simulink library "uavGuidanceForEachMod"  (R2021a)
settings: Solver=VariableStepAuto  StartTime=0.0  StopTime=10.0  RelTol=1e-3
undefined symbols (not defined in the file or in its folder): convertStringsToChars, initialState, m
settings Model: Creator=fciriell  LastModifiedBy=fciriell

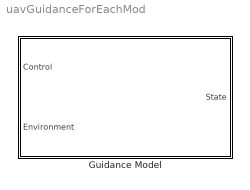
== system uavGuidanceForEachMod ==
  Guidance Model : Subsystem  mask(Guidance Model){ModelType=MultirotorGuidance, SpecifiedDataType=double, SimulateUsing=Code generation, InitialWorldPositionMultirotor=[0; 0; 0], InitialWorldVelocityMultirotor=[0; 0; 0], InitialEulerZYXMultirotor=[0; 0; 0], InitialBodyAngularRateRPYMultirotor=[0; 0; 0], InitialThrustMultirotor=0, InitialNorthFixedWing=0, InitialEastFixedWing=0, InitialHeightFixedWing=0, InitialAirSpeedFixedWing=0, InitialHeadingAngleFixedWing=0, InitialFlightPathAngleFixedWing=0, InitialRollAngleFixedWing=0, InitialRollAngleRateFixedWing=0, PDRollMultirotor=[3402.97,116.67], PDPitchMultirotor=[3402.97, 116.67], PYawRateMultirotor=1950, PThrustMultirotor=3900, MassMultirotor=m, PHeightFixedWing=3.9, PHeadingAngleFixedWing=3.9, PFlightPathAngleFixedWing=39, PDRollFixedWing=[3402.97, 116.67], PAirSpeedFixedWing=1, FlightPathAngleLimitsFixedWing=[-pi/2, pi/2], StateBusName='MultirotorGuidanceStateBus', ControlBusName='MultirotorGuidanceControlBus', EnvironmentBusName='MultirotorGuidanceEnvironmentBus', DataType=double}
      mask prompts: ModelType "uav:robotsluav:guidancemodelblock:ModelType"; SpecifiedDataType "uav:robotsluav:guidancemodelblock:DataType"; SimulateUsing "SystemBlock:MATLABSystem:SimulateUsing"; InitialWorldPositionMultirotor "uav:robotsluav:guidancemodelblock:WorldPosition"; InitialWorldVelocityMultirotor "uav:robotsluav:guidancemodelblock:WorldVelocity"; InitialEulerZYXMultirotor "uav:robotsluav:guidancemodelblock:EulerZYX"; InitialBodyAngularRateRPYMultirotor "uav:robotsluav:guidancemodelblock:BodyAngularRateRPY"; InitialThrustMultirotor "uav:robotsluav:guidancemodelblock:Thrust"; InitialNorthFixedWing "uav:robotsluav:guidancemodelblock:NorthPosition"; InitialEastFixedWing "uav:robotsluav:guidancemodelblock:EastPosition"; InitialHeightFixedWing "uav:robotsluav:guidancemodelblock:Height"; InitialAirSpeedFixedWing "uav:robotsluav:guidancemodelblock:AirSpeed"; InitialHeadingAngleFixedWing "uav:robotsluav:guidancemodelblock:HeadingAngle"; InitialFlightPathAngleFixedWing "uav:robotsluav:guidancemodelblock:FlightPathAngle"; InitialRollAngleFixedWing "uav:robotsluav:guidancemodelblock:RollAngle"; InitialRollAngleRateFixedWing "uav:robotsluav:guidancemodelblock:RollAngleRate"; PDRollMultirotor "uav:robotsluav:guidancemodelblock:PDRoll"; PDPitchMultirotor "uav:robotsluav:guidancemodelblock:PDPitch"; PYawRateMultirotor "uav:robotsluav:guidancemodelblock:PYawRate"; PThrustMultirotor "uav:robotsluav:guidancemodelblock:PThrust"; MassMultirotor "uav:robotsluav:guidancemodelblock:Mass"; PHeightFixedWing "uav:robotsluav:guidancemodelblock:PHeight"; PHeadingAngleFixedWing "uav:robotsluav:guidancemodelblock:PHeadingAngle"; PFlightPathAngleFixedWing "uav:robotsluav:guidancemodelblock:PFlightPathAngle"; PDRollFixedWing "uav:robotsluav:guidancemodelblock:PDRollAngle"; PAirSpeedFixedWing "uav:robotsluav:guidancemodelblock:PAirSpeed"; FlightPathAngleLimitsFixedWing "uav:robotsluav:guidancemodelblock:MinMaxFlightPathAngle"; StateBusName "uav:robotsluav:guidancemodelblock:StateBusName"; ControlBusName "uav:robotsluav:guidancemodelblock:ControlBusName"; EnvironmentBusName "uav:robotsluav:guidancemodelblock:EnvironmentBusName"; DataType "uav:robotsluav:guidancemodelblock:ResolvedDataType"
      mask help: uav:robotsluav:guidancemodelblock:Description
      mask init:
      | ModelName = gcb;
      | 
      | % Validate bus names
      | uav.sluav.internal.guidancemodel.mask.validateBusNames(gcb);
      | 
      | [stateDimension, initialState, UAVType, UAVDataType, UAVConfig] = ...
      |     uav.sluav.internal.guidancemodel.mask.initialize(ModelName, ModelType, gcb);
      mask Help: eval('helpview(fullfile(docroot, ''uav'', ''helptargets.map''), ''uavGuidanceModelBlock'')');
      mask TypeOptions ModelType: MultirotorGuidance | FixedWingGuidance
      mask Callback ModelType:
      | % Change mask dialog
      | uav.sluav.internal.guidancemodel.mask.modelTypeCallback(gcb);
      | 
      | % Create buses for the UAV block
      | uav.sluav.internal.guidancemodel.mask.createUAVBuses(gcb);
      mask Callback SpecifiedDataType:
      | if ~strcmp(get_param(gcb, 'SpecifiedDataType'), '<data type expression>')
      |     % Resolve input type
      |     uav.sluav.internal.guidancemodel.mask.dataTypeCallback(gcb);
      | 
      |     % Create buses for the UAV block
      |     uav.sluav.internal.guidancemodel.mask.createUAVBuses(gcb);
      | end
      mask TypeOptions SimulateUsing: ComputeDerivative/SimulateUsing | StateVector2Struct/SimulateUsing
      mask Callback StateBusName:
      | % Validate bus names
      | uav.sluav.internal.guidancemodel.mask.validateBusNames(gcb);
      | 
      | % Create buses for the UAV block
      | uav.sluav.internal.guidancemodel.mask.createUAVBuses(gcb);
      mask Callback ControlBusName:
      | % Validate bus names
      | uav.sluav.internal.guidancemodel.mask.validateBusNames(gcb);
      | 
      | % Create buses for the UAV block
      | uav.sluav.internal.guidancemodel.mask.createUAVBuses(gcb);
      mask Callback EnvironmentBusName:
      | % Validate bus names
      | uav.sluav.internal.guidancemodel.mask.validateBusNames(gcb);
      | 
      | % Create buses for the UAV block
      | uav.sluav.internal.guidancemodel.mask.createUAVBuses(gcb);
      mask DialogControl ModelType Prompt: Model Type:
      mask DialogControl SpecifiedDataType Prompt: Data Type:
      mask DialogControl SimulateUsing Prompt: Simulate using:
      mask DialogControl SimulateUsing Tooltip: SystemBlock:MATLABSystem:SimulateUsingDescription
      mask DialogControl InitialStateTab Prompt: uav:robotsluav:guidancemodelblock:InitialState
      mask DialogControl InitialWorldPositionMultirotor Prompt: World Position
      mask DialogControl InitialWorldVelocityMultirotor Prompt: World Velocity
      mask DialogControl InitialEulerZYXMultirotor Prompt: Euler Angles (ZYX)
      mask DialogControl InitialBodyAngularRateRPYMultirotor Prompt: Body Angular Rate
      mask DialogControl InitialThrustMultirotor Prompt: Thrust
      mask DialogControl InitialNorthFixedWing Prompt: North Position
      mask DialogControl InitialEastFixedWing Prompt: East Position
      mask DialogControl InitialHeightFixedWing Prompt: Height
      mask DialogControl InitialAirSpeedFixedWing Prompt: Air Speed
      mask DialogControl InitialHeadingAngleFixedWing Prompt: Heading Angle
      mask DialogControl InitialFlightPathAngleFixedWing Prompt: Flight Path Angle
      mask DialogControl InitialRollAngleFixedWing Prompt: Roll Angle
      mask DialogControl InitialRollAngleRateFixedWing Prompt: Roll Angular Velocity
      mask DialogControl ConfigurationTab Prompt: uav:robotsluav:guidancemodelblock:Configuration
      mask DialogControl PDRollMultirotor Prompt: PD Roll
      mask DialogControl PDPitchMultirotor Prompt: PD Pitch
      mask DialogControl PYawRateMultirotor Prompt: P YawRate
      mask DialogControl PThrustMultirotor Prompt: P Thrust
      mask DialogControl MassMultirotor Prompt: Mass
      mask DialogControl PHeightFixedWing Prompt: P Height
      mask DialogControl PHeadingAngleFixedWing Prompt: P Heading Angle
      mask DialogControl PFlightPathAngleFixedWing Prompt: P Flight Path Angle
      mask DialogControl PDRollFixedWing Prompt: PD Roll Angle
      mask DialogControl PAirSpeedFixedWing Prompt: P Air Speed
      mask DialogControl FlightPathAngleLimitsFixedWing Prompt: Min/Max Flight Path Angle
      mask DialogControl BusNameTab Prompt: uav:robotsluav:guidancemodelblock:InputOutputBusNames
      mask DialogControl StateBusName Prompt: State Bus Name
      mask DialogControl ControlBusName Prompt: Control Bus Name
      mask DialogControl EnvironmentBusName Prompt: Environment Bus Name
      mask DialogControl DataType Prompt: Resolved Data Type
      mask Display:
      | port_label('input', 1, 'Control')
      | port_label('input', 2, 'Environment')
      | port_label('output', 1, 'State')

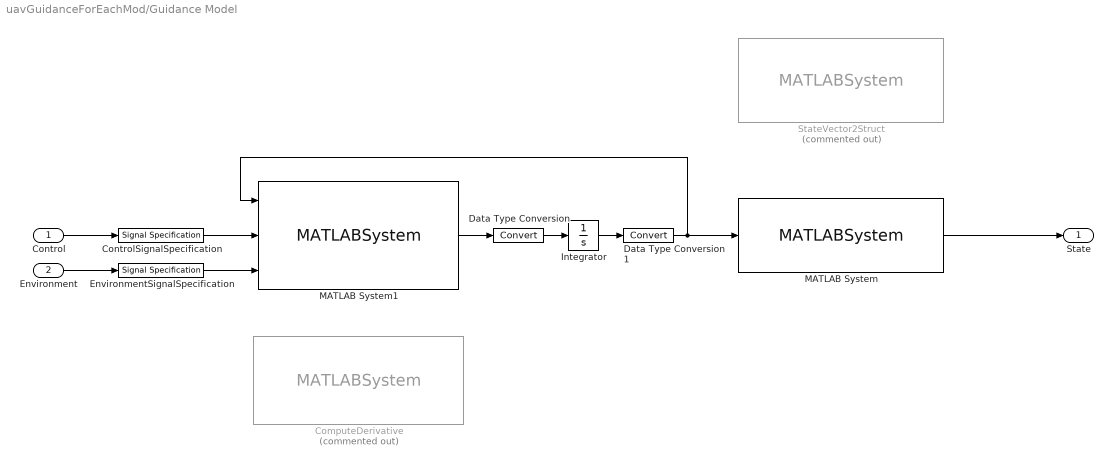
== system uavGuidanceForEachMod/Guidance Model ==
  Control : Inport
  Environment : Inport  Port=2
  ComputeDerivative : MATLABSystem  Commented=on  System=robotics.core.internal.system.navigation.Model  ModelName=ModelName  ModelType=UAVType  ModelConfiguration=UAVConfig  DataType=UAVDataType  UseExternalConfiguration=false  SimulateUsing=Code generation
      mask Type: robotics.core.internal.system.navigation.Model
      mask Display:
      | disp('Model');
      | port_label('input',1,'state');
      | port_label('input',2,'control');
      | port_label('input',3,'environment');
      | port_label('output',1,'stateDerivative');
  ControlSignalSpecification : SignalSpecification  OutDataTypeStr=Bus: MultirotorGuidanceControlBus  BusOutputAsStruct=on
  Data Type Conversion : DataTypeConversion
  Data Type Conversion1 : DataTypeConversion
  EnvironmentSignalSpecification : SignalSpecification  OutDataTypeStr=Bus: MultirotorGuidanceEnvironmentBus  BusOutputAsStruct=on
  Integrator : Integrator  InitialCondition=double(initialState)
  MATLAB System : MATLABSystem  System=StateVector2StructModForEach  OutputBusName=convertStringsToChars(StateBusName)  ModelType=UAVType  DataType=UAVDataType  SimulateUsing=Code generation
      mask Type: StateVector2StructModForEach
      mask Display:
      | disp('StateVector2StructModForEach');
      | port_label('input',1,'s');
      | port_label('output',1,'out');
  MATLAB System1 : MATLABSystem  System=ModelModForEach  ModelName=ModelName  ModelType=UAVType  ModelConfiguration=UAVConfig  DataType=UAVDataType  UseExternalConfiguration=false  SimulateUsing=Code generation
      mask Type: ModelModForEach
      mask Display:
      | disp('ModelModForEach');
      | port_label('input',1,'state');
      | port_label('input',2,'control');
      | port_label('input',3,'environment');
      | port_label('output',1,'stateDerivative');
  StateVector2Struct : MATLABSystem  Commented=on  System=robotics.core.internal.system.navigation.StateVector2Struct  OutputBusName=convertStringsToChars(StateBusName)  ModelType=UAVType  DataType=UAVDataType  SimulateUsing=Code generation
      mask Type: robotics.core.internal.system.navigation.StateVector2Struct
      mask Display:
      | disp('StateVector2Struct');
      | port_label('input',1,'s');
      | port_label('output',1,'out');
  State : Outport  VectorParamsAs1DForOutWhenUnconnected=off  BusOutputAsStruct=on
  wires:
  EnvironmentSignalSpecification/1 -> MATLAB System1/3
  ControlSignalSpecification/1 -> MATLAB System1/2
  Data Type Conversion1/1 -> MATLAB System1/1, MATLAB System/1
  Data Type Conversion/1 -> Integrator/1
  Environment/1 -> EnvironmentSignalSpecification/1
  Control/1 -> ControlSignalSpecification/1
  Integrator/1 -> Data Type Conversion1/1
  MATLAB System1/1 -> Data Type Conversion/1
  MATLAB System/1 -> State/1
